simulink model "MR-to-MP_simulation_system"  (R2019a)
settings: Solver=VariableStepAuto  StartTime=0.0  StopTime=720000  RelTol=1e-3
settings Model: Creator=86180  LastModifiedBy=86180

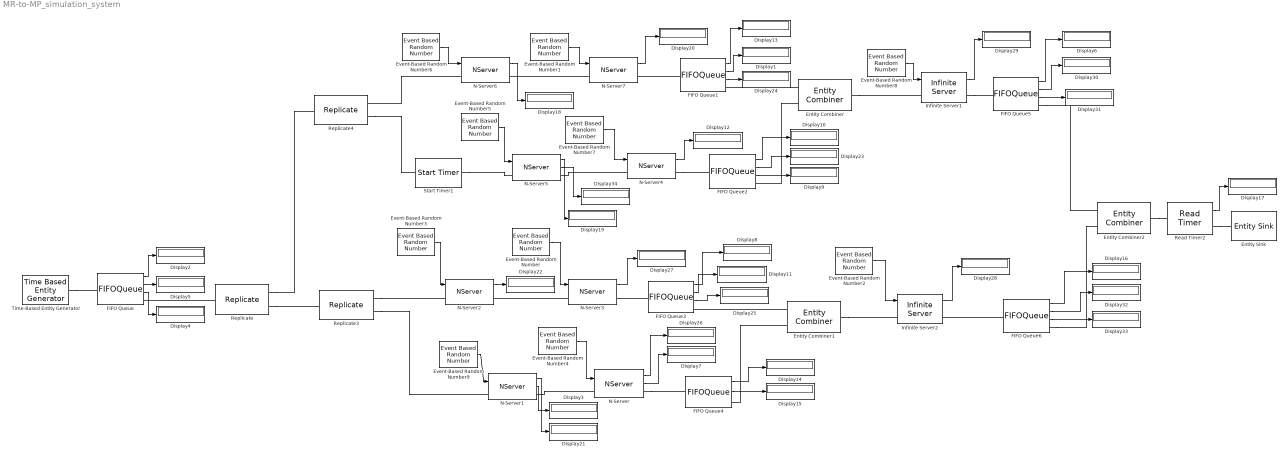
== system MR-to-MP_simulation_system ==
  Display{1..34} (34 alike) : Display
  Entity Combiner : EntityCombiner  NumberInputPorts=2  AttributeCopied=off
  Entity Combiner1 : EntityCombiner  NumberInputPorts=2  AttributeCopied=off
  Entity Combiner2 : EntityCombiner  NumberInputPorts=2  AttributeCopied=off
  Entity Sink : EntitySink
  Event-Based Random Number : EventBasedRandomNumber  meanExp=189  meanNorm=315  stdNorm=5  Seed=23578
  Event-Based Random Number1 : EventBasedRandomNumber  meanExp=189  meanNorm=315  stdNorm=5  Seed=30012
  Event-Based Random Number2 : EventBasedRandomNumber  meanExp=6  Seed=58140
  Event-Based Random Number3 : EventBasedRandomNumber  meanExp=6  meanNorm=12  stdNorm=3  Seed=53727
  Event-Based Random Number4 : EventBasedRandomNumber  meanExp=479  meanNorm=7  stdNorm=38  Seed=11535
  Event-Based Random Number5 : EventBasedRandomNumber  meanExp=7  meanNorm=7  stdNorm=38  Seed=14752
  Event-Based Random Number6 : EventBasedRandomNumber  meanExp=6  meanNorm=12  stdNorm=3  Seed=50510
  Event-Based Random Number7 : EventBasedRandomNumber  meanExp=479  meanNorm=7  stdNorm=38  Seed=17969
  Event-Based Random Number8 : EventBasedRandomNumber  meanExp=6  Seed=58965
  Event-Based Random Number9 : EventBasedRandomNumber  meanExp=7  meanNorm=7  stdNorm=38  Seed=24403
  FIFO Queue : FIFOQueue  Capacity=10000  StatNumberDeparted=on  StatAverageWait=on  StatAverageQueueLength=on
      settings: OutputPortMap=o0,o2,o3
  FIFO Queue1 : FIFOQueue  Capacity=1000  StatNumberDeparted=on  StatAverageWait=on  StatAverageQueueLength=on
      settings: OutputPortMap=o0,o2,o3
  FIFO Queue2 : FIFOQueue  Capacity=1000  StatNumberDeparted=on  StatAverageWait=on  StatAverageQueueLength=on
      settings: OutputPortMap=o0,o2,o3
  FIFO Queue3 : FIFOQueue  Capacity=1000  StatNumberDeparted=on  StatAverageWait=on  StatAverageQueueLength=on
      settings: OutputPortMap=o0,o2,o3
  FIFO Queue4 : FIFOQueue  Capacity=1000  StatAverageWait=on  StatAverageQueueLength=on
      settings: OutputPortMap=o2,o3
  FIFO Queue5 : FIFOQueue  StatNumberDeparted=on  StatAverageWait=on  StatAverageQueueLength=on
      settings: OutputPortMap=o0,o2,o3
  FIFO Queue6 : FIFOQueue  StatNumberDeparted=on  StatAverageWait=on  StatAverageQueueLength=on
      settings: OutputPortMap=o0,o2,o3
  Infinite Server1 : InfiniteServer  ServiceTimeFrom=Signal port t  StatAverageWait=on
      settings: OutputPortMap=o4
  Infinite Server2 : InfiniteServer  ServiceTimeFrom=Signal port t  StatAverageWait=on
      settings: OutputPortMap=o4
  N-Server : NServer  NumberOfServers=4  ServiceTimeFrom=Signal port t  StatAverageWait=on  StatUtilization=on
      settings: OutputPortMap=o4,o5
  N-Server1 : NServer  NumberOfServers=4  ServiceTimeFrom=Signal port t  StatAverageWait=on  StatUtilization=on
      settings: OutputPortMap=o4,o5
  N-Server2 : NServer  NumberOfServers=4  ServiceTimeFrom=Signal port t  StatAverageWait=on
      settings: OutputPortMap=o4
  N-Server3 : NServer  NumberOfServers=4  ServiceTimeFrom=Signal port t  StatAverageWait=on
      settings: OutputPortMap=o4
  N-Server4 : NServer  NumberOfServers=4  ServiceTimeFrom=Signal port t  StatUtilization=on
      settings: OutputPortMap=o5
  N-Server5 : NServer  NumberOfServers=4  ServiceTimeFrom=Signal port t  StatAverageWait=on  StatUtilization=on
      settings: OutputPortMap=o4,o5
  N-Server6 : NServer  NumberOfServers=4  ServiceTimeFrom=Signal port t  StatAverageWait=on
      settings: OutputPortMap=o4
  N-Server7 : NServer  NumberOfServers=4  ServiceTimeFrom=Signal port t  StatUtilization=on
      settings: OutputPortMap=o5
  Read Timer2 : ReadTimer  TimerTag=T2  StatAverageTimeElapsed=on
      settings: OutputPortMap=o3
  Replicate : Replicate  NumberOutputPorts=2
  Replicate3 : Replicate  NumberOutputPorts=2
  Replicate4 : Replicate  NumberOutputPorts=2
  Start Timer1 : StartTimer  TimerTag=T2
  Time-Based Entity Generator : TimeBasedEntityGenerator  Distribution=Exponential  InitialSeed=40859  Mean=3600/30
  wires:
  FIFO Queue/3 -> Display4/1
  FIFO Queue4/1 -> Display14/1
  Infinite Server2/1 -> Display28/1
  Event-Based Random Number2/1 -> Infinite Server2/1
  FIFO Queue/2 -> Display5/1
  Event-Based Random Number/1 -> N-Server3/1
  Event-Based Random Number3/1 -> N-Server2/1
  Event-Based Random Number4/1 -> N-Server/1
  FIFO Queue4/2 -> Display15/1
  FIFO Queue/1 -> Display2/1
  FIFO Queue3/1 -> Display8/1
  FIFO Queue3/2 -> Display11/1
  N-Server/2 -> Display7/1
  Event-Based Random Number6/1 -> N-Server6/1
  Event-Based Random Number1/1 -> N-Server7/1
  FIFO Queue1/2 -> Display1/1
  N-Server4/1 -> Display12/1
  FIFO Queue1/1 -> Display13/1
  Event-Based Random Number7/1 -> N-Server4/1
  Event-Based Random Number8/1 -> Infinite Server1/1
  Event-Based Random Number5/1 -> N-Server5/1
  Event-Based Random Number9/1 -> N-Server1/1
  Read Timer2/1 -> Display17/1
  FIFO Queue2/3 -> Display9/1
  FIFO Queue2/1 -> Display10/1
  N-Server7/1 -> Display20/1
  N-Server1/1 -> Display21/1
  N-Server6/1 -> Display18/1
  N-Server5/1 -> Display19/1
  N-Server2/1 -> Display22/1
  FIFO Queue2/2 -> Display23/1
  FIFO Queue1/3 -> Display24/1
  FIFO Queue3/3 -> Display25/1
  N-Server/1 -> Display26/1
  N-Server3/1 -> Display27/1
  Infinite Server1/1 -> Display29/1
  FIFO Queue6/1 -> Display16/1
  FIFO Queue5/1 -> Display6/1
  FIFO Queue5/2 -> Display30/1
  FIFO Queue5/3 -> Display31/1
  FIFO Queue6/2 -> Display32/1
  FIFO Queue6/3 -> Display33/1
  N-Server1/2 -> Display3/1
  N-Server5/2 -> Display34/1
  connections:
  FIFO Queue3/LConn1 -- N-Server3/RConn1
  Entity Combiner1/RConn1 -- Infinite Server2/LConn1
  N-Server3/LConn1 -- N-Server2/RConn1
  N-Server1/RConn1 -- N-Server/LConn1
  N-Server/RConn1 -- FIFO Queue4/LConn1
  N-Server7/LConn1 -- N-Server6/RConn1
  N-Server4/LConn1 -- N-Server5/RConn1
  Entity Combiner/LConn1 -- FIFO Queue1/RConn1
  N-Server4/RConn1 -- FIFO Queue2/LConn1
  FIFO Queue1/LConn1 -- N-Server7/RConn1
  Entity Combiner2/RConn1 -- Read Timer2/LConn1
  Replicate/LConn1 -- FIFO Queue/RConn1
  Entity Combiner/RConn1 -- Infinite Server1/LConn1
  Entity Combiner/LConn2 -- FIFO Queue2/RConn1
  Entity Combiner1/LConn1 -- FIFO Queue3/RConn1
  Entity Combiner1/LConn2 -- FIFO Queue4/RConn1
  Replicate/RConn1 -- Replicate4/LConn1
  Replicate3/RConn1 -- N-Server2/LConn1
  Replicate/RConn2 -- Replicate3/LConn1
  Replicate4/RConn2 -- Start Timer1/LConn1
  N-Server6/LConn1 -- Replicate4/RConn1
  Time-Based Entity Generator/RConn1 -- FIFO Queue/LConn1
  Read Timer2/RConn1 -- Entity Sink/LConn1
  Start Timer1/RConn1 -- N-Server5/LConn1
  Replicate3/RConn2 -- N-Server1/LConn1
  FIFO Queue5/RConn1 -- Entity Combiner2/LConn1
  FIFO Queue6/LConn1 -- Infinite Server2/RConn1
  FIFO Queue6/RConn1 -- Entity Combiner2/LConn2
  Infinite Server1/RConn1 -- FIFO Queue5/LConn1
